simulink model "W03_heading_control"  (R2024b)
settings: Solver=ode4  StartTime=0  StopTime=T_final  FixedStep=h  RelTol=1e-3
StopFcn:
  | W03_plot;
values from neighbouring files (symbols this model uses):
  animate = 1    [W03_0_setup.m]
  beta_c = 0    [W03_0_setup.m]
  c_d = 0    [W03_0_setup.m]
  h = 0.02    [W03_0_setup.m]    (also in W03_1_build_heading.m = Simulink.Annotation([m '/note']); W03_1_build_speed.m = add_line(sys, [a; via; b]); W03_1_build_surge_control.m = Simulink.Annotation([m '/note']); W03_H_build_antiwindup.m = Simulink.Annotation([sub '/how']))
  k_neg = cfg.k_neg    [W03_0_setup.m]
  k_pos = cfg.k_pos    [W03_0_setup.m]
  Kd = 74.90    (= 74.9)    [W03_0_setup.m]
  Kp = 100.00    (= 100)    [W03_0_setup.m]
  mp = 25    [W03_0_setup.m]
  n_max = cfg.n_max    [W03_0_setup.m]
  n_min = cfg.n_min    [W03_0_setup.m]
  psi_1 = 60    [W03_0_setup.m]
  psi_2 = 60    [W03_0_setup.m]
  rp = [0.05 0 -0.35]'    [W03_0_setup.m]
  t_dn = 1e6    (= 1000000)    [W03_0_setup.m]    (also in W03_animate.m = base_var('t_dn', inf))
  t_up = 5    [W03_0_setup.m]    (also in W03_animate.m = base_var('t_up', 0))
  use_ssa = 1    [W03_0_setup.m]
  V_c = 0    [W03_0_setup.m]
  x0 = zeros(12,1)    [W03_0_setup.m]
  X_ff = 60    [W03_0_setup.m]
  y_pont = cfg.y_pont    [W03_0_setup.m]
settings Model: Creator=admin  LastModifiedBy=admin
settings DataIOCC: ReturnWorkspaceOutputs=off

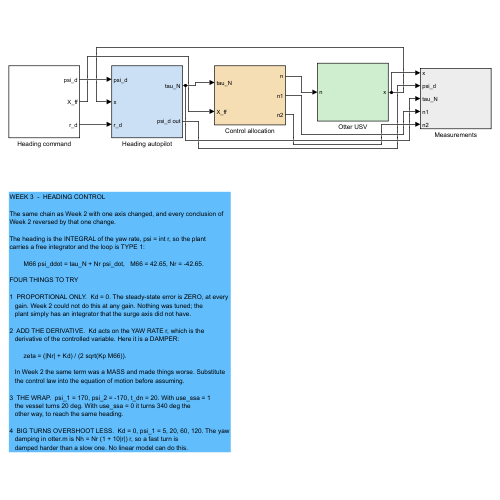
[thumbnail: Simulink's stored preview of the top-level diagram]
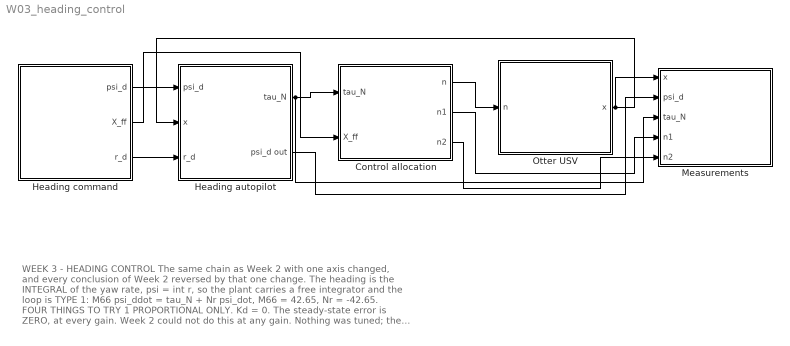
== system W03_heading_control ==
  note: WEEK 3  -  HEADING CONTROL
      |
      | The same chain as Week 2 with one axis changed, and every conclusion of
      | Week 2 reversed by that one change.
      |
      | The heading is the INTEGRAL of the yaw rate, psi = int r, so the plant
      | carries a free integrator and the loop is TYPE 1:
      |
      |         M66 psi_ddot = tau_N + Nr psi_dot,   M66 = 42.65, Nr = -42.65.
      |
      | FOUR THINGS TO TRY
      |
      | 1  PROPORTIONAL ONLY.  Kd = 0. The steady-state error is ZERO, at every
      |    gain. Week 2 could not do this at any gain. Nothing was tuned; the
      |    plant simply has an integrator that the surge axis did not have.
      |
      | 2  ADD THE DERIVATIVE.  Kd acts on the YAW RATE r, which is the
      |    derivative of the controlled variable. Here it is a DAMPER:
      |
      |         zeta = (|Nr| + Kd) / (2 sqrt(Kp M66)).
      |
      |    In Week 2 the same term was a MASS and made things worse. Substitute
      |    the control law into the equation of motion before assuming.
      |
      | 3  THE WRAP.  psi_1 = 170, psi_2 = -170, t_dn = 20. With use_ssa = 1
      |    the vessel turns 20 deg. With use_ssa = 0 it turns 340 deg the
      |    other way, to reach the same heading.
      |
      | 4  BIG TURNS OVERSHOOT LESS.  Kd = 0, psi_1 = 5, 20, 60, 120. The yaw
      |    damping in otter.m is Nh = Nr (1 + 10|r|) r, so a fast turn is
      |    damped harder than a slow one. No linear model can do this.
  Control allocation : Subsystem
  Heading autopilot : Subsystem
  Heading command : Subsystem
  Measurements : Subsystem
  Otter USV : Subsystem
  wires:
  Heading command/1(psi_d) -> Heading autopilot/1(psi_d)
  Otter USV/1(x) -> Heading autopilot/2(x), Measurements/1(x)
  Heading command/3(r_d) -> Heading autopilot/3(r_d)
  Heading autopilot/1(tau_N) -> Control allocation/1(tau_N), Measurements/3(tau_N)
  Heading command/2(X_ff) -> Control allocation/2(X_ff)
  Control allocation/1(n) -> Otter USV/1(n)
  Heading autopilot/2(psi_d out) -> Measurements/2(psi_d)
  Control allocation/2(n1) -> Measurements/4(n1)
  Control allocation/3(n2) -> Measurements/5(n2)

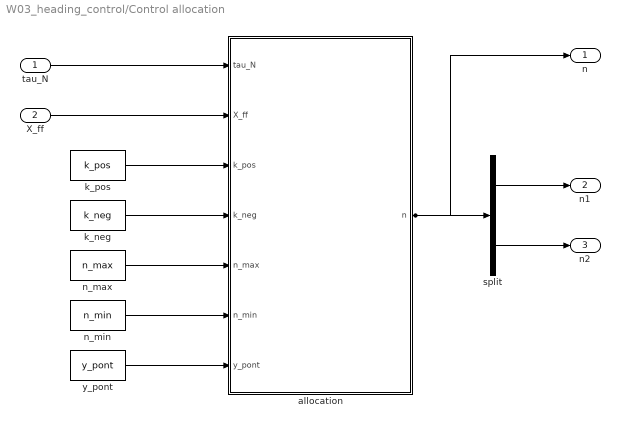
== system W03_heading_control/Control allocation ==
  tau_N : Inport
  X_ff : Inport  Port=2
  allocation : MATLAB Function  TreatAsAtomicUnit=on
  k_neg : Constant  Value=k_neg
  k_pos : Constant  Value=k_pos
  n_max : Constant  Value=n_max
  n_min : Constant  Value=n_min
  split : Demux  Outputs=2
  y_pont : Constant  Value=y_pont
  n : Outport
  n1 : Outport  Port=2
  n2 : Outport  Port=3
  wires:
  tau_N/1 -> allocation/1(tau_N)
  X_ff/1 -> allocation/2(X_ff)
  k_pos/1 -> allocation/3(k_pos)
  k_neg/1 -> allocation/4(k_neg)
  n_max/1 -> allocation/5(n_max)
  n_min/1 -> allocation/6(n_min)
  y_pont/1 -> allocation/7(y_pont)
  allocation/1(n) -> n/1, split/1
  split/1 -> n1/1
  split/2 -> n2/1

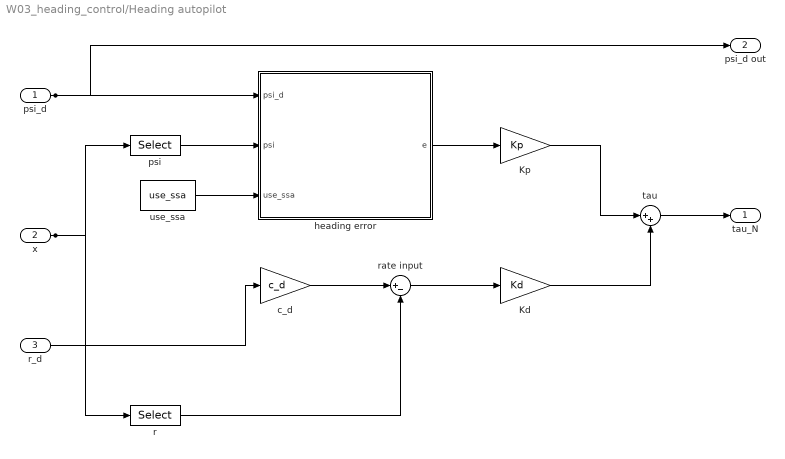
== system W03_heading_control/Heading autopilot ==
  psi_d : Inport
  x : Inport  Port=2
  r_d : Inport  Port=3
  Kd : Gain  Gain=Kd
  Kp : Gain  Gain=Kp
  c_d : Gain  Gain=c_d
  heading error : MATLAB Function  TreatAsAtomicUnit=on
  psi : Selector  InputPortWidth=12  IndexOptions=Index vector (dialog)  Indices=12  OutputSizes=1
  r : Selector  InputPortWidth=12  IndexOptions=Index vector (dialog)  Indices=6  OutputSizes=1
  rate input : Sum  Inputs=|+-
  tau : Sum  Inputs=|++
  use_ssa : Constant  Value=use_ssa
  tau_N : Outport
  psi_d out : Outport  Port=2
  wires:
  psi_d/1 -> heading error/1(psi_d), psi_d out/1
  psi/1 -> heading error/2(psi)
  use_ssa/1 -> heading error/3(use_ssa)
  x/1 -> psi/1, r/1
  heading error/1(e) -> Kp/1
  r_d/1 -> c_d/1
  c_d/1 -> rate input/1
  r/1 -> rate input/2
  rate input/1 -> Kd/1
  Kp/1 -> tau/1
  Kd/1 -> tau/2
  tau/1 -> tau_N/1

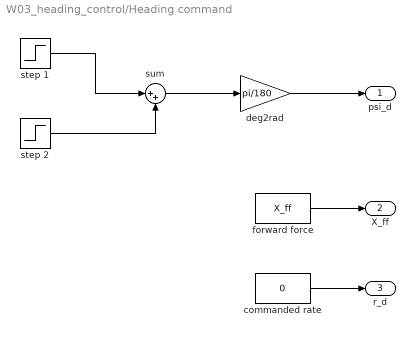
== system W03_heading_control/Heading command ==
  commanded rate : Constant  Value=0
  deg2rad : Gain  Gain=pi/180
  forward force : Constant  Value=X_ff
  step 1 : Step  Time=t_up  After=psi_1  SampleTime=0
  step 2 : Step  Time=t_dn  After=psi_2 - psi_1  SampleTime=0
  sum : Sum  Inputs=|++
  psi_d : Outport
  X_ff : Outport  Port=2
  r_d : Outport  Port=3
  wires:
  step 1/1 -> sum/1
  step 2/1 -> sum/2
  sum/1 -> deg2rad/1
  deg2rad/1 -> psi_d/1
  forward force/1 -> X_ff/1
  commanded rate/1 -> r_d/1

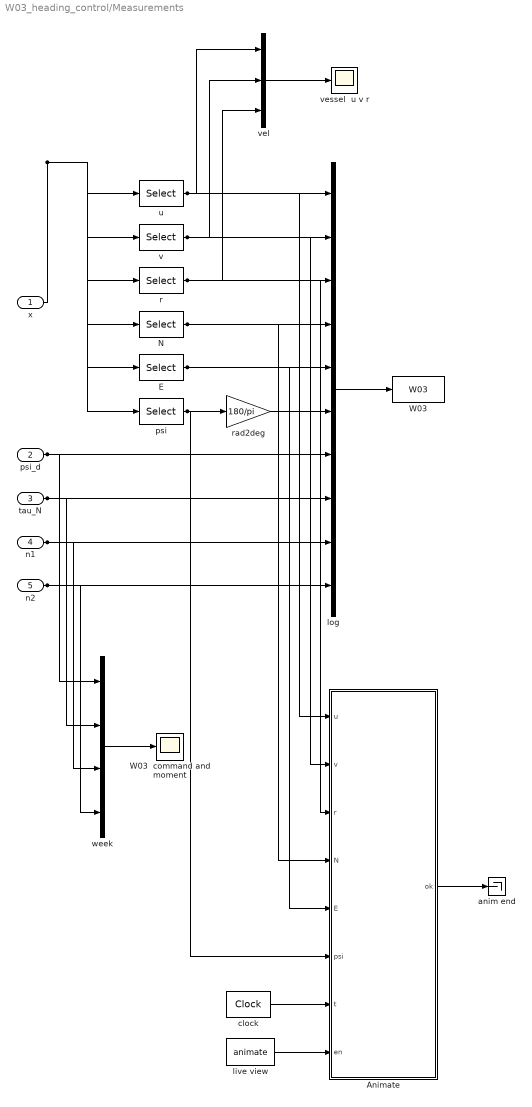
== system W03_heading_control/Measurements ==
  x : Inport
  psi_d : Inport  Port=2
  tau_N : Inport  Port=3
  n1 : Inport  Port=4
  n2 : Inport  Port=5
  Animate : MATLAB Function  TreatAsAtomicUnit=on
  E : Selector  InputPortWidth=12  IndexOptions=Index vector (dialog)  Indices=8  OutputSizes=1
  N : Selector  InputPortWidth=12  IndexOptions=Index vector (dialog)  Indices=7  OutputSizes=1
  W03 : ToWorkspace  VariableName=W03  SaveFormat=Structure With Time  SampleTime=-1
  W03  command and moment : Scope
  anim end : Terminator
  clock : DigitalClock  SampleTime=h
  live view : Constant  Value=animate
  log : Mux  Inputs=10
  psi : Selector  InputPortWidth=12  IndexOptions=Index vector (dialog)  Indices=12  OutputSizes=1
  r : Selector  InputPortWidth=12  IndexOptions=Index vector (dialog)  Indices=6  OutputSizes=1
  rad2deg : Gain  Gain=180/pi
  u : Selector  InputPortWidth=12  IndexOptions=Index vector (dialog)  Indices=1  OutputSizes=1
  v : Selector  InputPortWidth=12  IndexOptions=Index vector (dialog)  Indices=2  OutputSizes=1
  vel : Mux  Inputs=3
  vessel  u v r : Scope
  week : Mux
  wires:
  x/1 -> u/1, v/1, r/1, N/1, E/1, psi/1
  log/1 -> W03/1
  psi/1 -> rad2deg/1, Animate/6(psi)
  u/1 -> log/1, vel/1, Animate/1(u)
  v/1 -> log/2, vel/2, Animate/2(v)
  r/1 -> log/3, vel/3, Animate/3(r)
  N/1 -> log/4, Animate/4(N)
  E/1 -> log/5, Animate/5(E)
  rad2deg/1 -> log/6
  psi_d/1 -> log/7, week/1
  tau_N/1 -> log/8, week/2
  n1/1 -> log/9, week/3
  n2/1 -> log/10, week/4
  vel/1 -> vessel  u v r/1
  week/1 -> W03  command and moment/1
  clock/1 -> Animate/7(t)
  live view/1 -> Animate/8(en)
  Animate/1(ok) -> anim end/1

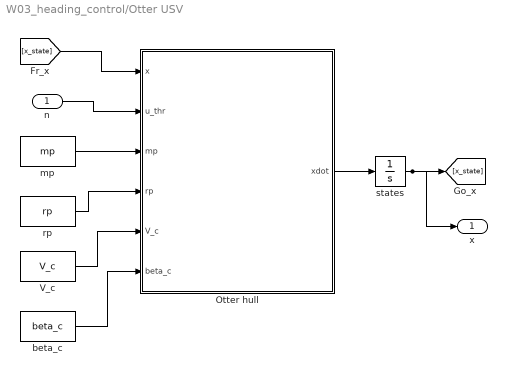
== system W03_heading_control/Otter USV ==
  n : Inport
  Otter hull : MATLAB Function  TreatAsAtomicUnit=on
  V_c : Constant  Value=V_c
  beta_c : Constant  Value=beta_c
  mp : Constant  Value=mp
  rp : Constant  Value=rp
  states : Integrator  InitialCondition=x0
  x : Outport
  wires:
  states/1 -> [x_state], x/1
  [x_state] -> Otter hull/1(x)
  Otter hull/1(xdot) -> states/1
  n/1 -> Otter hull/2(u_thr)
  beta_c/1 -> Otter hull/6(beta_c)
  rp/1 -> Otter hull/4(rp)
  mp/1 -> Otter hull/3(mp)
  V_c/1 -> Otter hull/5(V_c)

== matlab function W03_heading_control/Control allocation/allocation ==
  data: tau_N input; n output double size=[2 1]; X_ff input; k_pos input; k_neg input; n_max input; n_min input; y_pont input
function n = allocation(tau_N, X_ff, k_pos, k_neg, n_max, n_min, y_pont)
%#codegen
% Demanded surge force and yaw moment to two shaft speeds.
%
% Step 1, the exact inverse of tau = B f:
%     T1 = X/2 + N/(2 y_pont)
%     T2 = X/2 - N/(2 y_pont)
%
% Step 2, the propeller curve inverted one propeller at a time:
%     n = sign(T) sqrt(|T| / k),  with k_pos ahead and k_neg astern.
%
% Allocating THRUST and inverting afterwards is what makes the two shaft
% speeds come out unequal by themselves. A pure yaw moment gives T2 = -T1,
% and because k_neg < k_pos the reverse shaft must turn faster. Appendix A1
% derives that pair by hand; here it falls out of the arithmetic.
T = [X_ff/2 + tau_N/(2*y_pont);
     X_ff/2 - tau_N/(2*y_pont)];
n = zeros(2,1);
for i = 1:2
    if T(i) >= 0
        ni =  sqrt( T(i) / k_pos);
    else
        ni = -sqrt(-T(i) / k_neg);
    end
    n(i) = min(max(ni, n_min), n_max);
end
end

== matlab function W03_heading_control/Heading autopilot/heading error ==
  data: psi_d input; e output double size=[1 1]; psi input; use_ssa input
function e = headingerror(psi_d, psi, use_ssa)
%#codegen
% Smallest signed angle between two headings.
%
%   ssa(a) maps any angle into (-pi, pi], so the controller always turns the
%   SHORT way round. Without it, a command of -170 deg while heading +170 deg
%   reads as an error of -340 deg and the vessel turns almost all the way
%   round to reach a heading 20 deg away.
%
% use_ssa = 0 removes the wrap, which is the experiment of section E.
e = psi_d - psi;
if use_ssa > 0.5
    e = atan2(sin(e), cos(e));
end
end

== matlab function W03_heading_control/Otter USV/Otter hull ==
  data: x input; xdot output double size=[12 1]; u_thr input; mp input; rp input; V_c input; beta_c input
function xdot = otter_hull(x, u_thr, mp, rp, V_c, beta_c)
% Fossen's otter.m, called unchanged from Tools/MSS/VESSELS.
%
%   x       12 states, fed back from the integrator
%   u_thr   propeller shaft speeds [rad/s]
%
% otter.m is not written for code generation, so the call is extrinsic and
% xdot has to be pre-sized for Simulink to know the output width.
coder.extrinsic('otter');

xdot = zeros(12,1);
xdot = otter(x, u_thr, mp, rp, V_c, beta_c);
end

== matlab function W03_heading_control/Measurements/Animate ==
  data: u input; ok output; v input; r input; N input; E input; psi input; t input; en input
function ok = Animate(u, v, r, N, E, psi, t, en)
%#codegen
% Live view of the vessel while the model runs.
%
% A MATLAB Function block cannot plot, so the drawing function is declared
% extrinsic: Simulink calls plain MATLAB rather than generating code for it.
% Set animate = 0 in the setup script to switch the live view off.
%
% psi arrives in RADIANS and r in rad/s - the units otter.m works in. The
% wrapper converts them for display, in one place, so no two figures in the
% course can disagree about what a degree is.
coder.extrinsic('W03_animate');
ok = 1;
if en > 0.5
    W03_animate(u, v, r, N, E, psi, t);
end
end
